simulink model "payload_6dof"  (R2024b)
settings: configuration reference "prj_default_config" (kept outside this file)
settings Model: Creator=yangyu  LastModifiedBy=yangyu
settings ConfigSetRef: SourceName=prj_default_config  SourceLocation=Base Workspace

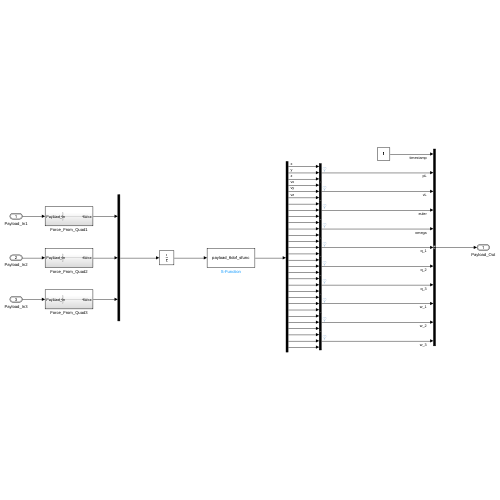
[thumbnail: Simulink's stored preview of the top-level diagram]
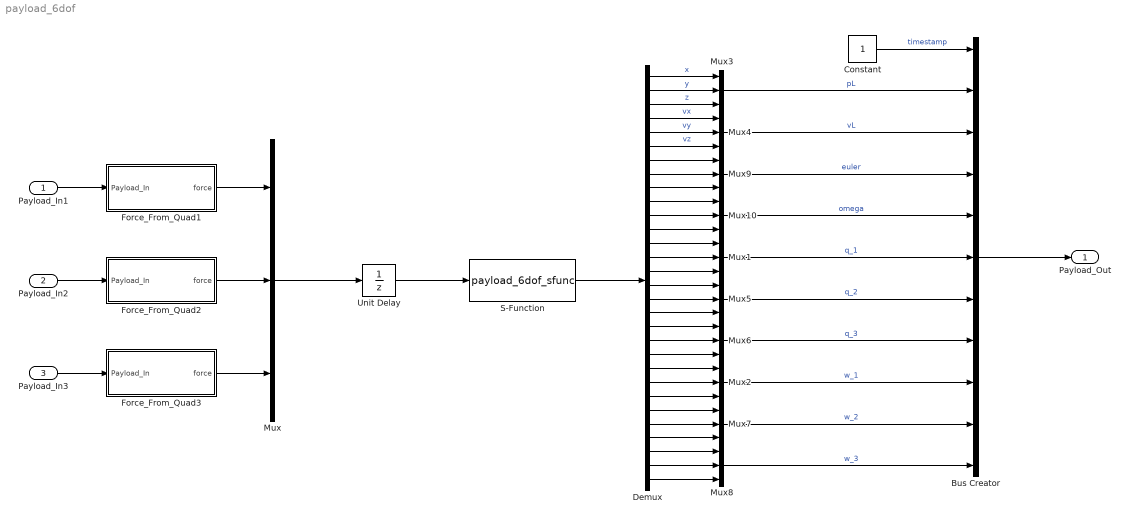
== system payload_6dof ==
  Payload_In1 : Inport  OutDataTypeStr=Bus: Payload_In_Bus
  Payload_In2 : Inport  Port=2  OutDataTypeStr=Bus: Payload_In_Bus
  Payload_In3 : Inport  Port=3  OutDataTypeStr=Bus: Payload_In_Bus
  Bus Creator : BusCreator  Inputs=11  OutDataTypeStr=Bus: Payload_Out_Bus
  Constant : Constant  OutDataTypeStr=Inherit: Inherit via back propagation
  Demux : Demux  Outputs=30
  Force_From_Quad1 : Subsystem
  Force_From_Quad2 : Subsystem
  Force_From_Quad3 : Subsystem
  Mux{,1..10} (11 alike) : Mux  Inputs=3
  S-Function : S-Function  FunctionName=payload_6dof_sfunc  SFunctionDeploymentMode=off  EnableBusSupport=off
  Unit Delay : UnitDelay  SampleTime=-1  HasFrameUpgradeWarning=on
  Payload_Out : Outport  OutDataTypeStr=Bus: Payload_Out_Bus
  wires:
  S-Function/1 -> Demux/1
  Demux/1 -> Mux3/1  "x"
  Demux/2 -> Mux3/2  "y"
  Demux/3 -> Mux3/3  "z"
  Force_From_Quad1/1(force) -> Mux/1
  Demux/4 -> Mux4/1  "vx"
  Demux/5 -> Mux4/2  "vy"
  Demux/6 -> Mux4/3  "vz"
  Force_From_Quad2/1(force) -> Mux/2
  Force_From_Quad3/1(force) -> Mux/3
  Mux3/1 -> Bus Creator/2  "pL"
  Mux4/1 -> Bus Creator/3  "vL"
  Payload_In1/1 -> Force_From_Quad1/1(Payload_In)
  Payload_In2/1 -> Force_From_Quad2/1(Payload_In)
  Payload_In3/1 -> Force_From_Quad3/1(Payload_In)
  Constant/1 -> Bus Creator/1  "timestamp"
  Bus Creator/1 -> Payload_Out/1
  Mux/1 -> Unit Delay/1
  Unit Delay/1 -> S-Function/1
  Demux/15 -> Mux1/3
  Demux/27 -> Mux7/3
  Mux2/1 -> Bus Creator/9  "w_1"
  Mux5/1 -> Bus Creator/7  "q_2"
  Demux/24 -> Mux2/3
  Demux/29 -> Mux8/2
  Demux/22 -> Mux2/1
  Demux/19 -> Mux6/1
  Mux6/1 -> Bus Creator/8  "q_3"
  Demux/21 -> Mux6/3
  Demux/16 -> Mux5/1
  Demux/26 -> Mux7/2
  Mux8/1 -> Bus Creator/11  "w_3"
  Mux1/1 -> Bus Creator/6  "q_1"
  Mux7/1 -> Bus Creator/10  "w_2"
  Demux/14 -> Mux1/2
  Demux/13 -> Mux1/1
  Demux/17 -> Mux5/2
  Demux/25 -> Mux7/1
  Demux/20 -> Mux6/2
  Demux/18 -> Mux5/3
  Demux/23 -> Mux2/2
  Demux/30 -> Mux8/3
  Demux/28 -> Mux8/1
  Demux/8 -> Mux9/2
  Demux/9 -> Mux9/3
  Demux/7 -> Mux9/1
  Mux9/1 -> Bus Creator/4  "euler"
  Demux/11 -> Mux10/2
  Demux/10 -> Mux10/1
  Demux/12 -> Mux10/3
  Mux10/1 -> Bus Creator/5  "omega"

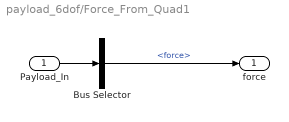
== system payload_6dof/Force_From_Quad1 ==
  Payload_In : Inport
  Bus Selector : BusSelector  OutputSignals=force
  force : Outport
  wires:
  Payload_In/1 -> Bus Selector/1
  Bus Selector/1 -> force/1  "<force>"

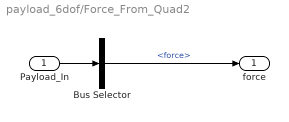
== system payload_6dof/Force_From_Quad2 ==
  Payload_In : Inport
  Bus Selector : BusSelector  OutputSignals=force
  force : Outport
  wires:
  Bus Selector/1 -> force/1  "<force>"
  Payload_In/1 -> Bus Selector/1

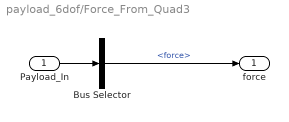
== system payload_6dof/Force_From_Quad3 ==
  Payload_In : Inport
  Bus Selector : BusSelector  OutputSignals=force
  force : Outport
  wires:
  Payload_In/1 -> Bus Selector/1
  Bus Selector/1 -> force/1  "<force>"
